simulink model "sim_mcce_scheduled_control_saved"  (R2016a)
settings: Solver=VariableStepAuto  StartTime=0.0  StopTime=0.5  RelTol=1e-5
undefined symbols (not defined in the file): Ad_lt, Bd_lt, Cd_lt, DiscIntNeverNeededParam, Kdi_lt, Kdo_lt, Ts, ws_lt
settings Model: Creator=manuel  LastModifiedBy=manuel

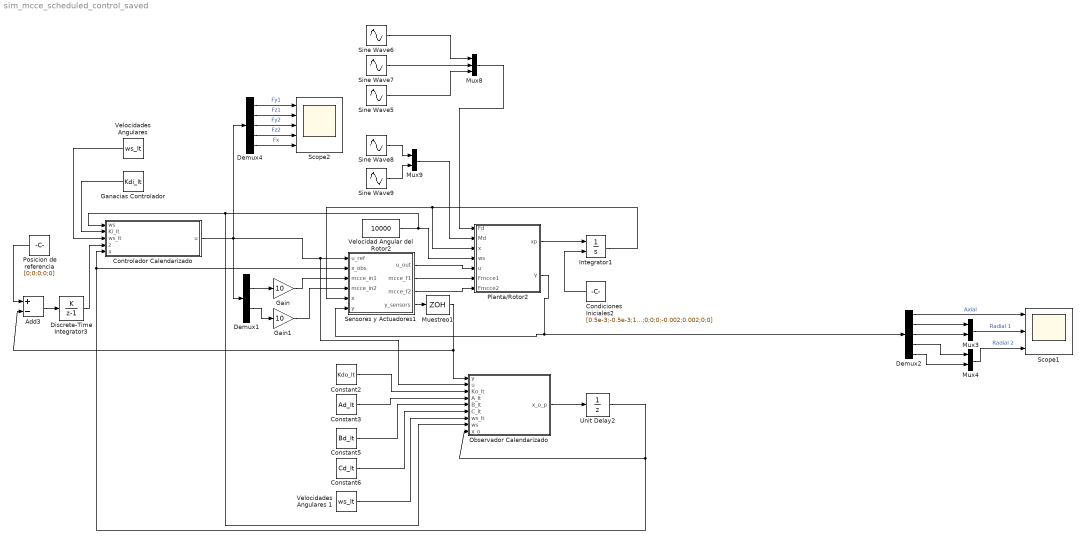
== system sim_mcce_scheduled_control_saved ==
  Add3 : Sum  Inputs=+-
  Condiciones Iniciales2 : Constant  Value=[0.5e-3;-0.5e-3;1e-3;0;0;0;-0.002;0.002;0;0]
  Constant2 : Constant  Value=Kdo_lt  VectorParams1D=off
  Constant3 : Constant  Value=Ad_lt  VectorParams1D=off
  Constant5 : Constant  Value=Bd_lt  VectorParams1D=off
  Constant6 : Constant  Value=Cd_lt  VectorParams1D=off
  Controlador Calendarizado : MATLAB Function  TreatAsAtomicUnit=on
  Demux1 : Demux  Outputs=5
  Demux2 : Demux  Outputs=5
  Demux4 : Demux  Outputs=5
  Discrete-Time Integrator3 : DiscreteIntegrator  IntegratorMethod=Accumulation: Forward Euler  gainval=1  InitialCondition=[0;0;0;0;0]  InitialConditionSetting=State (most efficient)  SampleTime=-1  ICPrevOutput=DiscIntNeverNeededParam  ICPrevScaledInput=DiscIntNeverNeededParam
  Gain : Gain  Gain=10
  Gain1 : Gain  Gain=10
  Ganacias Controlador : Constant  Value=Kdi_lt  VectorParams1D=off
  Integrator1 : Integrator  InitialConditionSource=external  InitialCondition=[0;0;0;0;0;0;0;0;0;0]
  Muestreo1 : ZeroOrderHold  SampleTime=Ts
  Mux3 : Mux  Inputs=2
  Mux4 : Mux  Inputs=2
  Mux8 : Mux  Inputs=3
  Mux9 : Mux  Inputs=2
  Observador Calendarizado : MATLAB Function  TreatAsAtomicUnit=on
  Planta/Rotor2 : MATLAB Function  TreatAsAtomicUnit=on
  Posicion de referencia : Constant  Value=[0;0;0;0;0]
  Scope1 : Scope  NumInputPorts=3
  Scope2 : Scope  NumInputPorts=5
  Sensores y Actuadores1 : Subsystem
  Sine Wave5 : Sin  Amplitude=3  Bias=10  Frequency=100*2*pi  SampleTime=0
  Sine Wave6 : Sin  Frequency=50*2*pi  SampleTime=0
  Sine Wave7 : Sin  Frequency=100*2*pi  SampleTime=0
  Sine Wave8 : Sin  Amplitude=0  Frequency=600*2*pi  SampleTime=0
  Sine Wave9 : Sin  Amplitude=0  Frequency=300*2*pi  SampleTime=0
  Unit Delay2 : UnitDelay  InitialCondition=[0;0;0;0;0;0;0;0;0;0]  SampleTime=-1
  Velocidad Angular del Rotor2 : Constant  Value=10000  VectorParams1D=off
  Velocidades Angulares : Constant  Value=ws_lt  VectorParams1D=off
  Velocidades Angulares 1 : Constant  Value=ws_lt  VectorParams1D=off
  wires:
  ? -> ?
  Demux2/2 -> Mux3/1
  Demux2/3 -> Mux3/2
  Demux2/4 -> Mux4/1
  Demux2/5 -> Mux4/2
  Mux3/1 -> Scope1/2  "Radial 1"
  Mux4/1 -> Scope1/3  "Radial 2"
  Demux4/1 -> Scope2/1  "Fy1"
  Demux4/2 -> Scope2/2  "Fz1"
  Demux4/3 -> Scope2/3  "Fy2"
  Demux4/4 -> Scope2/4  "Fz2"
  Demux4/5 -> Scope2/5  "Fx"
  Demux2/1 -> Scope1/1  "Axial"
  Ganacias Controlador/1 -> Controlador Calendarizado/2(Ki_lt)
  Constant2/1 -> Observador Calendarizado/3(Ko_lt)
  Constant3/1 -> Observador Calendarizado/4(A_lt)
  Constant5/1 -> Observador Calendarizado/5(B_lt)
  Constant6/1 -> Observador Calendarizado/6(C_lt)
  Velocidades Angulares/1 -> Controlador Calendarizado/3(ws_lt)
  Velocidades Angulares 1/1 -> Observador Calendarizado/7(ws_lt)
  Integrator1/1 -> Sensores y Actuadores1/5(x), Planta/Rotor2/3(x)
  Planta/Rotor2/1(xp) -> Integrator1/1
  Posicion de referencia/1 -> Add3/1
  Unit Delay2/1 -> Observador Calendarizado/9(x_o), Sensores y Actuadores1/2(x_obs), Controlador Calendarizado/5(x)
  Gain/1 -> Sensores y Actuadores1/3(mcce_in1)
  Gain1/1 -> Sensores y Actuadores1/4(mcce_in2)
  Sensores y Actuadores1/1(u_out) -> Planta/Rotor2/5(u)
  Sensores y Actuadores1/2(mcce_f1) -> Planta/Rotor2/6(Fmcce1)
  Sensores y Actuadores1/3(mcce_f2) -> Planta/Rotor2/7(Fmcce2)
  Planta/Rotor2/2(y) -> Sensores y Actuadores1/6(y), Demux2/1
  Sensores y Actuadores1/4(y_sensors) -> Muestreo1/1
  Condiciones Iniciales2/1 -> Integrator1/2
  Muestreo1/1 -> Observador Calendarizado/1(y), Add3/2
  Add3/1 -> Discrete-Time Integrator3/1
  Observador Calendarizado/1(x_o_p) -> Unit Delay2/1
  Discrete-Time Integrator3/1 -> Controlador Calendarizado/4(z)
  Velocidad Angular del Rotor2/1 -> Controlador Calendarizado/1(ws), Observador Calendarizado/8(ws), Planta/Rotor2/4(ws)
  Demux1/2 -> Gain/1
  Demux1/4 -> Gain1/1
  Controlador Calendarizado/1(u) -> Observador Calendarizado/2(u), Sensores y Actuadores1/1(u_ref), Demux4/1, Demux1/1
  Mux9/1 -> Planta/Rotor2/2(Md)
  Mux8/1 -> Planta/Rotor2/1(Fd)
  Sine Wave8/1 -> Mux9/1
  Sine Wave9/1 -> Mux9/2
  Sine Wave7/1 -> Mux8/2
  Sine Wave5/1 -> Mux8/3
  Sine Wave6/1 -> Mux8/1

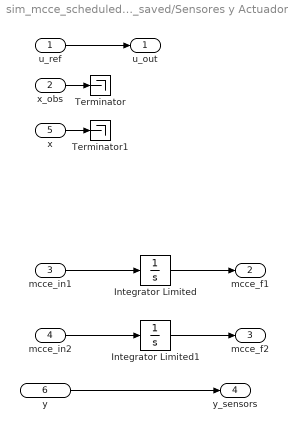
== system sim_mcce_scheduled_control_saved/Sensores y Actuadores1 ==
  u_ref : Inport
  x_obs : Inport  Port=2
  mcce_in1 : Inport  Port=3
  mcce_in2 : Inport  Port=4
  x : Inport  Port=5
  y : Inport  Port=6
  Integrator Limited : Integrator  InitialCondition=6  LimitOutput=on  UpperSaturationLimit=40  LowerSaturationLimit=6
  Integrator Limited1 : Integrator  InitialCondition=6  LimitOutput=on  UpperSaturationLimit=40  LowerSaturationLimit=6
  Terminator : Terminator
  Terminator1 : Terminator
  u_out : Outport
  mcce_f1 : Outport  Port=2
  mcce_f2 : Outport  Port=3
  y_sensors : Outport  Port=4
  wires:
  y/1 -> y_sensors/1
  x/1 -> Terminator1/1
  Integrator Limited1/1 -> mcce_f2/1
  mcce_in2/1 -> Integrator Limited1/1
  mcce_in1/1 -> Integrator Limited/1
  Integrator Limited/1 -> mcce_f1/1
  x_obs/1 -> Terminator/1
  u_ref/1 -> u_out/1

== matlab function sim_mcce_scheduled_control_saved/Observador Calendarizado ==
  data: y input; u input; x_o_p output; Ko_lt input; A_lt input; B_lt input; C_lt input; ws_lt input; ws input; x_o input
function x_o_p = state_obsever(y,u,Ko_lt,A_lt,B_lt,C_lt,ws_lt,ws,x_o)
%#codegen
Ko = matrix_interpolation(ws_lt,Ko_lt,ws);
A = matrix_interpolation(ws_lt,A_lt,ws);
B = matrix_interpolation(ws_lt,B_lt,ws);
C = matrix_interpolation(ws_lt,C_lt,ws);

x_o_p = A*x_o + B*u + Ko*(y-C*x_o);

== matlab function sim_mcce_scheduled_control_saved/Planta//Rotor2 ==
  data: Fd input; Md input; xp output; x input; ws input; y output; u input; Fmcce1 input; Fmcce2 input
function [xp,y]  = fcn(Fd,Md,x,ws,u,Fmcce1,Fmcce2)
Fd_x = Fd(1);
Fd_y = Fd(2);
Fd_z = Fd(3);
Md_y = Md(1);
Md_z = Md(2);
[xp,y] = hmb_non_linear_model(x,u,ws,Fd_x,Fd_y,Fd_z,Md_y,Md_z,Fmcce1,Fmcce2);
end

== matlab function sim_mcce_scheduled_control_saved/Controlador Calendarizado ==
  data: ws input; Ki_lt input; ws_lt input; z input; x input; u output
function u  = feedback_controller(ws,Ki_lt,ws_lt,z,x)
%#codegen
ki = matrix_interpolation(ws_lt,Ki_lt,ws);

xi = [x;z];

u = -ki*xi;
